simulink model "sf_mandelbrot_fixpt"  (Simulink 7.6)
settings: Solver=FixedStepDiscrete  SolverMode=SingleTasking  StartTime=0.0  StopTime=inf  FixedStep=0.0005  RelTol=1e-3
CloseFcn:
  | sf_mandel_gui('close');
settings Model: Creator=The MathWorks Inc.  CovMetricSettings=dcmtr  ExtModeAutoUpdateStatusClock=off
settings DataIOCC: SaveOutput=off  SaveTime=off
settings OptimizationCC: BooleanDataType=off  InitFltsAndDblsToZero=on  EfficientMapNaN2IntZero=off  BufferReusableBoundary=off
settings DebuggingCC: SignalResolutionControl=TryResolveAllWithWarning  SolverPrmCheckMsg=none  MultiTaskDSMMsg=warning  MultiTaskCondExecSysMsg=none  BusObjectLabelMismatch=none  StrictBusMsg=None
settings HardwareCC: TargetUnknown=on
settings SFSimCC: SFSimEcho=off  SimParseCustomCode=off
settings RTWCC: IncludeERTFirstTime=on
settings GRTTargetCC: TargetFcnLib=ansi_tfl_tmw.mat

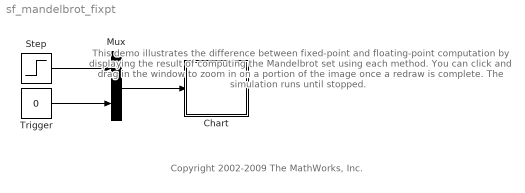
== system sf_mandelbrot_fixpt ==
  note: This demo illustrates the difference between
      | fixed-point and floating-point computation by
      | displaying the result of computing the
      | Mandelbrot set using each method.
      |
      | You can click and drag in the window to zoom
      | in on a portion of the image once a redraw is
      | complete. The simulation runs until stopped.
  note: Copyright 2002-2009 The MathWorks, Inc.
  Chart : Stateflow chart  TreatAsAtomicUnit=on
  Mux : Mux  Inputs=2
  Step : Step  Time=0.1  SampleTime=0  ZeroCross=off
  Trigger : Constant  Value=0
  wires:
  Trigger/1 -> Mux/2
  Step/1 -> Mux/1
  Mux/1 -> Chart/Trigger

== stateflow chart Chart ==
  state ii = mandel_fix(a0,b0) [function]
    (default) -> (junction 6) : { ii = 0;
        |  r2 = 0;
        |  local_colors = colors; }
    (junction 6) -> (junction 7) : {
        | bn = 2 * an * bn + b0;
        | an = r2 + a0;
        | r2 = an * an - bn * bn;
        | }
    (junction 11) -> (junction 8) : {
        | ii++;
        | }
    (junction 8) -> (junction 6)
    (junction 7) -> (junction 9) [order 2]
    (junction 7) -> (junction 11) [order 1] : [ r2 < 4 && ii < local_colors ]
  state Wait
    entry:ml.sf_mandel_gui("enter_wait");
  state ii = mandel_double(a0,b0) [function]
    (junction 20) -> (junction 22) [order 1] : [ r2 < 4 && ii < local_colors ]
    (junction 20) -> (junction 18) [order 2]
    (junction 19) -> (junction 21)
    (junction 22) -> (junction 19) : {
        | ii++;
        | }
    (junction 21) -> (junction 20) : {
        | bn = 2 * an * bn + b0;
        | an = r2 + a0;
        | r2 = an * an - bn * bn;
        | }
    (default) -> (junction 21) : { ii = 0;
        |  r2 = 0;
        |  local_colors = colors; }
  (junction 15) -> Wait [order 2] : { ml.toc() }
  (junction 17) -> (junction 10) : {
      | fix_line[j]  = mandel_fix(x,y0);
      | dbl_line[j] = mandel_double(x,y0);
      | }
  (junction 10) -> (junction 12)
  (junction 12) -> (junction 13) : {
      | j++;
      | x += deltax;
      | }
  (default) -> (junction 14) : {
      | ml.sf_mandel_gui();
      | }
  (junction 23) -> (junction 15)
  (junction 15) -> (junction 16) [order 1] : [ i <= pix_h ]
  (junction 16) -> (junction 17) : {
      | j = 1;
      | x = real_left;
      | }
  (junction 13) -> (junction 17) [order 1] : [ j <= pix_w]
  (junction 13) -> (junction 15) [order 2] : {
      | ml.sf_mandel_gui(i,dbl_line,fix_line);
      | ml.sf_mandel_gui("update");
      | i++;
      | y0 -= deltay;
      | }
  (junction 14) -> (junction 23) : {
      | ml.sf_mandel_gui("exit_wait");
      | colors = ml.sf_mandel_gui("colors");
      |
      | pix_w = ml.sf_mandel_gui("pixel width");
      | pix_h  = ml.sf_mandel_gui("pixel height");
      |
      | real_left = ml.sf_mandel_gui("real left");
      | real_top = ml.sf_mandel_gui("real top");
      | real_w   = ml.sf_mandel_gui("real width");
      | real_h   = ml.sf_mandel_gui("real height");
      |
      | deltax = real_w / pix_w;
      | deltay = real_h / pix_h;
      |
      | i=1;
      | y0 = real_top;
      | ml.tic();
      | }
  Wait -> (junction 14) : Redraw
  data: a0 function_input fixdt(1,16,13); b0 function_input fixdt(1,16,13); an temporary fixdt(1,16,13); bn temporary fixdt(1,16,13); ii function_output int32; r2 temporary fixdt(1,32,26); local_colors temporary int32; a0 function_input double; b0 function_input double; an temporary double; bn temporary double; ii function_output int32; local_colors temporary int32; r2 temporary double; real_left local double; real_w local double; pix_w local double; deltax local double; deltay local double; i local int32; y0 local double; j local int32; x local double; real_top local double; real_h local double; pix_h local double; colors local double; fix_line local double size=1024; dbl_line local double size=1024
  events: Start input EITHER_EDGE_EVENT; Redraw input EITHER_EDGE_EVENT
